simulink model "Lights"  (R2021a)
settings: Solver=FixedStepDiscrete  StartTime=0.0  StopTime=60.0  FixedStep=0.1  RelTol=1e-3
settings Model: EnablePacing=on  Creator=ncleju  LastModifiedBy=ncleju

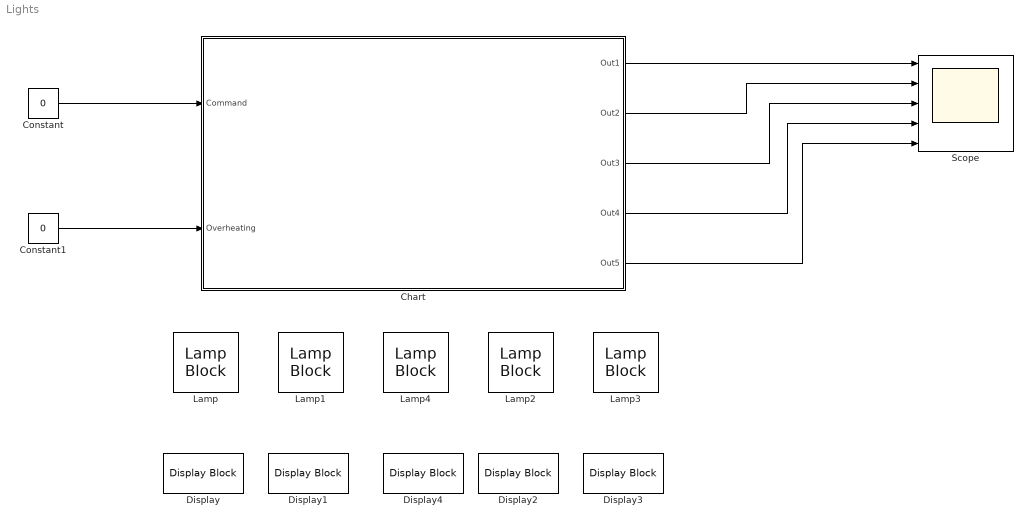
== system Lights ==
  Chart : Stateflow chart  TreatAsAtomicUnit=on
  Constant : Constant  Value=0
  Constant1 : Constant  Value=0
  Display{,1..4} (5 alike) : DisplayBlock  LabelPosition=Hide  Format=short  Transparency=1
  Lamp{,1..4} (5 alike) : LampBlock
  Scope : Scope  NumInputPorts=5
  wires:
  Chart/1(Out1) -> Scope/1
  Chart/2(Out2) -> Scope/2
  Chart/3(Out3) -> Scope/3
  Chart/4(Out4) -> Scope/4
  Chart/5(Out5) -> Scope/5
  Constant/1 -> Chart/1(Command)
  Constant1/1 -> Chart/2(Overheating)

== stateflow chart Lights/Chart ==
  state NORMAL
    (history)
    state MODE2
      state INCREASING
        en:
        Out1 = 0;
        Out2 = 0;
        Out3 = 0;
        Out4 = 0;
        Out5 = 0;
        du:
        Out1 = Out1 + 3.33;
        Out2 = Out2 + 3.33;
        Out3 = Out3 + 3.33;
        Out4 = Out4 + 3.33;
        Out5 = Out5 + 3.33;
      state DECREASING
        en:
        Out1 = 100;
        Out2 = 100;
        Out3 = 100;
        Out4 = 100;
        Out5 = 100;
        du:
        Out1 = Out1 - 3.33;
        Out2 = Out2 - 3.33;
        Out3 = Out3 - 3.33;
        Out4 = Out4 - 3.33;
        Out5 = Out5 - 3.33;
      (default) -> INCREASING
      INCREASING -> DECREASING : [after(3, sec)]
      DECREASING -> INCREASING : [[after(3, sec)]]
    state MODE1
      state ON
        en:
        Out1 = 100;
        Out2 = 100;
        Out3 = 100;
        Out4 = 100;
        Out5 = 100;
      state OFF
        en:
        Out1 = 0;
        Out2 = 0;
        Out3 = 0;
        Out4 = 0;
        Out5 = 0;
      (default) -> ON
      ON -> OFF : [after(200, msec)]
      OFF -> ON : [after(200, msec)]
    state MODE3
      state TRAIN1
        en:
        Out1 = 100;
        Out2 = 0;
        Out3 = 0;
        Out4 = 0;
        Out5 = 0;
      state TRAIN2
        en:
        Out1 = 0;
        Out2 = 100;
        Out3 = 0;
        Out4 = 0;
        Out5 = 0;
      state TRAIN3
        en:
        Out1 = 0;
        Out2 = 0;
        Out3 = 100;
        Out4 = 0;
        Out5 = 0;
      state TRAIN4
        en:
        Out1 = 0;
        Out2 = 0;
        Out3 = 0;
        Out4 = 100;
        Out5 = 0;
      state TRAIN5
        en:
        Out1 = 0;
        Out2 = 0;
        Out3 = 0;
        Out4 = 0;
        Out5 = 100;
      (default) -> TRAIN1
      TRAIN4 -> TRAIN5 : [after(300, msec)]
      TRAIN1 -> TRAIN2 : [after(300, msec)]
      TRAIN2 -> TRAIN3 : [after(300, msec)]
      TRAIN3 -> TRAIN4 : [after(300, msec)]
      TRAIN5 -> (junction 43) : [after(300, msec)]
      (junction 43) -> (junction 44)
      (junction 46) -> TRAIN1
      (junction 45) -> (junction 46)
      (junction 44) -> (junction 45)
    (default) -> MODE1
    MODE1 -> MODE2 [order 1] : [after(10, sec) && Command == 0]
    MODE2 -> MODE1 [order 2] : [Command == 1]
    MODE1 -> MODE2 [order 2] : [Command == 2]
    MODE1 -> MODE3 [order 3] : [Command == 3]
    MODE2 -> MODE3 [order 3] : [Command == 3]
    MODE2 -> MODE3 [order 1] : [after(12, sec)  && Command == 0]
    MODE3 -> MODE2 [order 3] : [Command == 2]
    MODE3 -> MODE1 [order 2] : [Command == 1]
    MODE3 -> MODE1 [order 1] : [after(10, sec) && Command == 0]
  state OVERHEATING
    en:
    Out1 = 0;
    Out2 = 0;
    Out3 = 0;
    Out4 = 0;
    Out5 = 0;
  (default) -> NORMAL
  NORMAL -> OVERHEATING : [Overheating == true]
  OVERHEATING -> NORMAL : [Overheating == false && after(15, sec)]
  data: Out1 output; Out2 output; Out3 output; Out4 output; Out5 output; Command input; Overheating input
